simulink model "sampleModel295"  (R2021b)
settings: Solver=VariableStepAuto  StartTime=0.0  StopTime=10.0  RelTol=1e-3
undefined symbols (not defined in the file or in its folder): Newton, Raphson
libraries: simulink x10, slpidlib x2
settings Model: Creator=user  LastModifiedBy=user

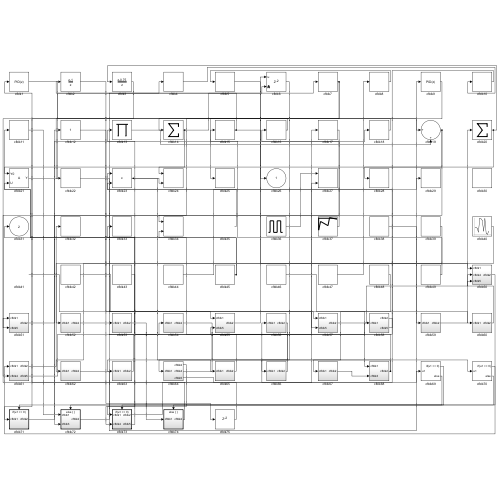
[thumbnail: Simulink's stored preview of the top-level diagram]
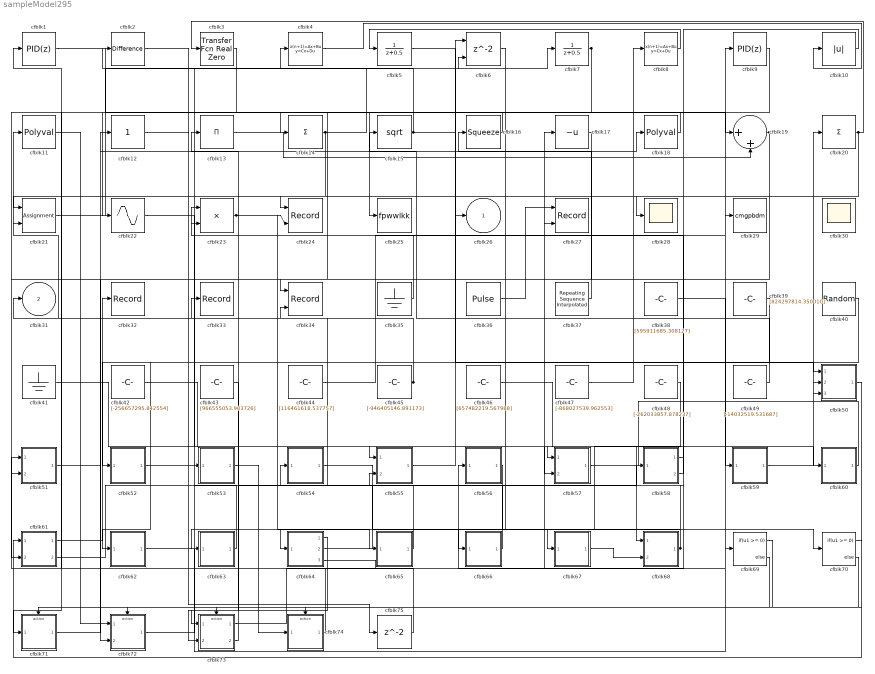
== system sampleModel295 ==
  cfblk1 : slpidlib/PID Controller  Controller=PID  Form=Parallel  TimeDomain=Discrete-time  UseExternalTs=off  SampleTime=1  IntegratorMethod=Forward Euler  FilterMethod=Forward Euler  ControllerParametersSource=internal  P=1  I=1  D=0  UseFilter=on  N=100  TunerSelectOption=Transfer Function Based (PID Tuner App)  InitialConditionSource=internal  InitialConditionForIntegrator=0  InitialConditionForFilter=0  DifferentiatorICPrevScaledInput=0  ExternalReset=none  TrackingMode=off  Kt=1  LimitOutput=off  SatLimitsSource=internal  UpperSaturationLimit=inf  LowerSaturationLimit=-inf  LinearizeAsGain=off  AntiWindupMode=none  Kb=1  POutMin=[]  POutMax=[]  IOutMin=[]  IOutMax=[]  DOutMin=[]  DOutMax=[]  NOutMin=[]  NOutMax=[]  SumOutMin=[]  SumOutMax=[]  SaturationOutMin=[]  SaturationOutMax=[]  PParamMin=[]  PParamMax=[]  IParamMin=[]  IParamMax=[]  DParamMin=[]  DParamMax=[]  NParamMin=[]  NParamMax=[]  KbParamMin=[]  KbParamMax=[]  KtParamMin=[]  KtParamMax=[]  KbOutMin=[]  KbOutMax=[]  KtOutMin=[]  KtOutMax=[]  IntegratorOutMin=[]  IntegratorOutMax=[]  FilterOutMin=[]  FilterOutMax=[]  SumI1OutMin=[]  SumI1OutMax=[]  SumI2OutMin=[]  SumI2OutMax=[]  SumI3OutMin=[]  SumI3OutMax=[]  SumI4OutMin=[]  SumI4OutMax=[]  SumDOutMin=[]  SumDOutMax=[]  DifferentiatorOutMin=[]  DifferentiatorOutMax=[]  FilterDiffOutCoefMin=[]  FilterDiffOutCoefMax=[]  ReciprocalOutMin=[]  ReciprocalOutMax=[]  SumDenOutMin=[]  SumDenOutMax=[]  SumNumOutMin=[]  SumNumOutMax=[]  DivideOutMin=[]  DivideOutMax=[]  UdiffTsProdOutMin=[]  UdiffTsProdOutMax=[]  NTsProdOutMin=[]  NTsProdOutMax=[]  UintegralTsProdOutMin=[]  UintegralTsProdOutMax=[]  UngainTsProdOutMin=[]  UngainTsProdOutMax=[]  IntegratorContinuousStateAttributes=''  IntegratorStateMustResolveToSignalObject=off  IntegratorRTWStateStorageClass=Auto  FilterContinuousStateAttributes=''  FilterStateMustResolveToSignalObject=off  FilterRTWStateStorageClass=Auto  ParallelPVariant=InternalParameters  IdealPVariant=Disabled  IVariant=InternalParameters  DVariant=InternalParameters  IntegratorVariant=Discrete  SatVariant=Disabled  AWVariant=Passthrough  PCopyVariant=Disabled  TRVariant=Disabled  FdbkBlocksVariant=Forward  IdealPFdbkVariant=Disabled  SatFdbkVariant=Disabled  DerivativeFilterVariant=ForwardEulerFilter  NVariant=InternalParameters  NCopyVariant=Disabled  FilterICVariant=InternalICsFilter  IntegratorICVariant=InternalICs  ExternalResetVariant=Disabled  TRSumVariant=Passthrough  SumFdbkVariant=Disabled  SumVariant=Sum_PID  TsampFilterVariant=InternalTs  TsampNgainVariant=Passthrough  TsampIntegralVariant=Passthrough  ExternalSaturationOutDataTypeStr=Inherit: Same as second input
  cfblk10 : Abs
  cfblk11 : Polyval  Coefs=[ +2.081618890e-019, -1.441693666e-014, +4.719686976e-010, -8.536869453e-006, +1.621573104e-001, -8.087801117e+001 ]
  cfblk12 : simulink/Math Operations/Slider Gain  gain=1  low=0  high=2
  cfblk13 : Product  Inputs=*
  cfblk14 : Sum  Inputs=+
  cfblk15 : Sqrt  SaturateOnIntegerOverflow=on
  cfblk16 : Squeeze
  cfblk17 : UnaryMinus
  cfblk18 : Polyval  Coefs=[ +2.081618890e-019, -1.441693666e-014, +4.719686976e-010, -8.536869453e-006, +1.621573104e-001, -8.087801117e+001 ]
  cfblk19 : Sum  Inputs=|++
  cfblk2 : simulink/Discrete/Difference  ICPrevInput=0.0  OutMin=[]  OutMax=[]  OutDataTypeStr=Inherit: Inherit via back propagation  OutDataType=fixdt(1, 16)  OutScaling=2^-10  DoSatur=off
  cfblk20 : Sum  Inputs=+
  cfblk21 : Assignment  DiagnosticForDimensions=Warning  IndexOptions=Index vector (dialog)  Indices=1  OutputSizes=1
  cfblk22 : Sin  TimeSource=Use external signal  SampleTime=0
  cfblk23 : Product  Inputs=**
  cfblk24 : Record  FileSettingsInternal="{\"entries\":[{\"content\":{\"excelSettings\":{\"content\":{},\"type\":\"Streamout.ExcelSettings\"}},\"type\":\"Streamout.FileSettingStorage\",\"uuid\":\"e644294e-47c8-4157-a70f-b86bf0f91ce5\"}],\"packageUris\":[\"http://schema.mathworks.com/mf0/streamout_blocks/R2020a\"],\"version\":\"1.0\"}"  Layout=[1 1]  SignalsInternal="{\"entries\":[{\"content\":{\"signals\":[{\"content\":{\"blockPath\":[\"sampleModel295/cfblk24\"],\"channel\":[],\"dimensions\":[1],\"domain\":\"sampleModel295/cfblk24\",\"lineColor\":\"#a2142f\",\"plots\":[1],\"port\":1,\"sid\":[\"\"],\"signalID\":12729,\"signalName\":\"cfblk14\"},\"type\":\"RecordBlkView.Signal\",\"uuid\":\"f10aec68-513e-477d-a584-377b7a0421ce\"},{\"content\":{\"blockPath\":[\"sampleModel295/cfblk24\"],\"channel\":[],\"dimensions\":[1,1],\"domain\":\"sampleModel295/cfblk24\",\"lineColor\":\"#139fff\",\"plots\":[1],\"port\":2,\"sid\":[\"\"],\"signalID\":12733,\"signalName\":\"cfblk23\"},\"type\":\"RecordBlkView.Signal\",\"uuid\":\"9a725780-6232-41e5-9a59-fff5a766301b\"}]},\"type\":\"RecordBlkView.InputSignals\",\"uuid\":\"3815a519-980c-4b72-ad09-c02e00f9a3ac\"}],\"packageUris\":[\"http://schema.mathworks.com/mf0/streamout_blocks/R2020a\"],\"version\":\"1.0\"}"  VisualizationBindings="{\"xyplotplugin\":{\"info\":[{\"series\":[{\"bindingParametersList\":[{\"parameter\":\"X-Axis\",\"signalID\":12729,\"signalName\":\"cfblk14\"},{\"parameter\":\"Y-Axis\",\"signalID\":12733,\"signalName\":\"cfblk23\"}],\"seriesID\":57202}],\"subplotID\":1}]}}"  CompatibilityTag=XY
  cfblk25 : ToWorkspace  VariableName=fpwwlkk  SaveFormat=Timeseries  SampleTime=-1
  cfblk27 : Record  FileSettingsInternal="{\"entries\":[{\"content\":{\"excelSettings\":{\"content\":{},\"type\":\"Streamout.ExcelSettings\"}},\"type\":\"Streamout.FileSettingStorage\",\"uuid\":\"b7e32862-4def-4129-82f2-dd9595ad73df\"}],\"packageUris\":[\"http://schema.mathworks.com/mf0/streamout_blocks/R2020a\"],\"version\":\"1.0\"}"  Layout=[1 1]  SignalsInternal="{\"entries\":[{\"content\":{\"signals\":[{\"content\":{\"blockPath\":[\"sampleModel295/cfblk27\"],\"channel\":[],\"dimensions\":[1],\"domain\":\"sampleModel295/cfblk27\",\"lineColor\":\"#a2142f\",\"plots\":[1],\"port\":1,\"sid\":[\"\"],\"signalID\":12737,\"signalName\":\"cfblk36\"},\"type\":\"RecordBlkView.Signal\",\"uuid\":\"85d272bf-6785-403c-95ae-8b25dcc783db\"},{\"content\":{\"blockPath\":[\"sampleModel295/cfblk27\"],\"channel\":[],\"dimensions\":[1],\"domain\":\"sampleModel295/cfblk27\",\"lineColor\":\"#139fff\",\"plots\":[1],\"port\":2,\"sid\":[\"\"],\"signalID\":12741,\"signalName\":\"cfblk73:1\"},\"type\":\"RecordBlkView.Signal\",\"uuid\":\"b5cff7ce-ee06-4cac-90c4-86c035636aeb\"}]},\"type\":\"RecordBlkView.InputSignals\",\"uuid\":\"7b9cfb08-aa55-403e-a887-71b5e0abc4a4\"}],\"packageUris\":[\"http://schema.mathworks.com/mf0/streamout_blocks/R2020a\"],\"version\":\"1.0\"}"  VisualizationBindings="{\"xyplotplugin\":{\"info\":[{\"series\":[{\"bindingParametersList\":[{\"parameter\":\"X-Axis\",\"signalID\":12737,\"signalName\":\"cfblk36\"},{\"parameter\":\"Y-Axis\",\"signalID\":12741,\"signalName\":\"cfblk73:1\"}],\"seriesID\":37411}],\"subplotID\":1}]}}"  CompatibilityTag=XY
  cfblk28 : Scope
  cfblk29 : ToWorkspace  VariableName=cmgpbdm  SaveFormat=Timeseries  SampleTime=-1
  cfblk3 : simulink/Discrete/Transfer Fcn Real Zero  ZeroZ=0.75  ICPrevInput=0.0  DoSatur=off
      settings: SourceProductBaseCode=SL
  cfblk30 : Scope
      settings: Floating=on
  cfblk32 : Record  FileSettingsInternal="{\"entries\":[{\"content\":{\"excelSettings\":{\"content\":{},\"type\":\"Streamout.ExcelSettings\"}},\"type\":\"Streamout.FileSettingStorage\",\"uuid\":\"9b634011-b706-471f-8d8c-3277855acf29\"}],\"packageUris\":[\"http://schema.mathworks.com/mf0/streamout_blocks/R2020a\"],\"version\":\"1.0\"}"  SignalsInternal="{\"entries\":[{\"content\":{\"signals\":[{\"content\":{\"blockPath\":[\"sampleModel295/cfblk32\"],\"channel\":[],\"dimensions\":[1],\"domain\":\"sampleModel295/cfblk32\",\"lineColor\":\"#a2142f\",\"plots\":[1],\"port\":1,\"sid\":[\"\"],\"signalID\":12745,\"signalName\":\"cfblk61:1\"},\"type\":\"RecordBlkView.Signal\",\"uuid\":\"713a4e37-51c4-4904-a6cc-f5381fe626eb\"}]},\"type\":\"RecordBlkView.InputSignals\",\"uuid\":\"94e50211-0dd7-4ae3-a9db-9c1dd3a17ac5\"}],\"packageUris\":[\"http://schema.mathworks.com/mf0/streamout_blocks/R2020a\"],\"version\":\"1.0\"}"  VisualizationBindings="{\"sparklinesplugin\":{\"info\":[{\"bindingParametersList\":[],\"subplotID\":1}]}}"
  cfblk33 : Record  FileSettingsInternal="{\"entries\":[{\"content\":{\"excelSettings\":{\"content\":{},\"type\":\"Streamout.ExcelSettings\"}},\"type\":\"Streamout.FileSettingStorage\",\"uuid\":\"9bcf9a1a-6272-4e85-9a14-13b62b86e8eb\"}],\"packageUris\":[\"http://schema.mathworks.com/mf0/streamout_blocks/R2020a\"],\"version\":\"1.0\"}"  SignalsInternal="{\"entries\":[{\"content\":{\"signals\":[{\"content\":{\"blockPath\":[\"sampleModel295/cfblk33\"],\"channel\":[],\"dimensions\":[1,1],\"domain\":\"sampleModel295/cfblk33\",\"lineColor\":\"#139fff\",\"plots\":[1],\"port\":1,\"sid\":[\"\"],\"signalID\":12749,\"signalName\":\"cfblk65\"},\"type\":\"RecordBlkView.Signal\",\"uuid\":\"4cbff2d7-f26b-4c35-8c5f-df1d9d9f7d13\"}]},\"type\":\"RecordBlkView.InputSignals\",\"uuid\":\"b3f169fd-622d-4759-a4e5-6eade6133a40\"}],\"packageUris\":[\"http://schema.mathworks.com/mf0/streamout_blocks/R2020a\"],\"version\":\"1.0\"}"  VisualizationBindings="{\"sparklinesplugin\":{\"info\":[{\"bindingParametersList\":[],\"subplotID\":1}]}}"
  cfblk34 : Record  FileSettingsInternal="{\"entries\":[{\"content\":{\"excelSettings\":{\"content\":{},\"type\":\"Streamout.ExcelSettings\"}},\"type\":\"Streamout.FileSettingStorage\",\"uuid\":\"ad245534-a126-491f-ae91-c836af0e3ad9\"}],\"packageUris\":[\"http://schema.mathworks.com/mf0/streamout_blocks/R2020a\"],\"version\":\"1.0\"}"  Layout=[1 1]  SignalsInternal="{\"entries\":[{\"content\":{\"signals\":[{\"content\":{\"blockPath\":[\"sampleModel295/cfblk34\"],\"channel\":[],\"dimensions\":[1],\"domain\":\"sampleModel295/cfblk34\",\"lineColor\":\"#a2142f\",\"plots\":[1],\"port\":1,\"sid\":[\"\"],\"signalID\":12753,\"signalName\":\"cfblk7\"},\"type\":\"RecordBlkView.Signal\",\"uuid\":\"bce65451-ca10-46cc-b2c4-c9a99149bc20\"},{\"content\":{\"blockPath\":[\"sampleModel295/cfblk34\"],\"channel\":[],\"dimensions\":[1,1],\"domain\":\"sampleModel295/cfblk34\",\"lineColor\":\"#139fff\",\"plots\":[1],\"port\":2,\"sid\":[\"\"],\"signalID\":12757,\"signalName\":\"cfblk68\"},\"type\":\"RecordBlkView.Signal\",\"uuid\":\"bca2518a-e4c1-488f-a659-4f0ad251d5cd\"}]},\"type\":\"RecordBlkView.InputSignals\",\"uuid\":\"252255dc-c8db-4030-b98c-8f428237fd4d\"}],\"packageUris\":[\"http://schema.mathworks.com/mf0/streamout_blocks/R2020a\"],\"version\":\"1.0\"}"  VisualizationBindings="{\"xyplotplugin\":{\"info\":[{\"series\":[{\"bindingParametersList\":[{\"parameter\":\"X-Axis\",\"signalID\":12753,\"signalName\":\"cfblk7\"},{\"parameter\":\"Y-Axis\",\"signalID\":12757,\"signalName\":\"cfblk68\"}],\"seriesID\":47423}],\"subplotID\":1}]}}"  CompatibilityTag=XY
  cfblk35 : Ground
  cfblk36 : DiscretePulseGenerator  PulseType=Time based  Amplitude=[-849674981.811508]  Period=[1552871.382462]  PulseWidth=5  PhaseDelay=[8.000000]
  cfblk37 : simulink/Sources/Repeating Sequence Interpolated  OutValues=[-984002673.050901, -258940035.022713, -628170089.492454, 59276096.145658, -75844292.440838]  TimeValues=[0 0.1 0.5 0.6 1].'  LookUpMeth=Use Input Nearest  tsamp=0.01  OutMin=[]  OutMax=[]  OutDataTypeStr=double  OutputDataTypeScalingMode=double  OutDataType=fixdt(0,8)  OutScaling=2^-10
  cfblk38 : Constant  Value=[595911685.308127]  SampleTime=1
  cfblk39 : Constant  Value=[824297814.350010]  SampleTime=1
  cfblk4 : DiscreteStateSpace
  cfblk40 : RandomNumber  Mean=[37993.970635]  Variance=[6255.361900]  Seed=[560915355.000000]  SampleTime=0.1
  cfblk41 : Ground
  cfblk42 : Constant  Value=[-256657295.842554]  SampleTime=1
  cfblk43 : Constant  Value=[966555053.903726]  SampleTime=1
  cfblk44 : Constant  Value=[116461618.537757]  SampleTime=1
  cfblk45 : Constant  Value=[-946405146.891173]  SampleTime=1
  cfblk46 : Constant  Value=[657482219.567988]  SampleTime=1
  cfblk47 : Constant  Value=[-868027539.962553]  SampleTime=1
  cfblk48 : Constant  Value=[-262033857.878237]  SampleTime=1
  cfblk49 : Constant  Value=[-14032519.531687]  SampleTime=1
  cfblk5 : DiscreteTransferFcn  SampleTime=1
  cfblk50 : Subsystem
  cfblk51 : Subsystem
  cfblk52 : Subsystem
  cfblk53 : Subsystem
  cfblk54 : Subsystem
  cfblk55 : Subsystem
  cfblk56 : Subsystem
  cfblk57 : Subsystem
  cfblk58 : Subsystem
  cfblk59 : Subsystem
  cfblk6 : Delay  ShowEnablePort=on  SampleTime=1
      settings: InputPortMap=u0,e6
  cfblk60 : Subsystem
  cfblk61 : Subsystem
  cfblk62 : Subsystem
  cfblk63 : Subsystem
  cfblk64 : Subsystem
  cfblk65 : Subsystem
  cfblk66 : Subsystem
  cfblk67 : Subsystem
  cfblk68 : Subsystem
  cfblk69 : If  IfExpression=u1 >= 0  SampleTime=1
  cfblk7 : DiscreteTransferFcn  SampleTime=1
  cfblk70 : If  IfExpression=u1 >= 0  SampleTime=1
  cfblk71 : Subsystem  TreatAsAtomicUnit=on
  cfblk72 : Subsystem  TreatAsAtomicUnit=on
  cfblk73 : Subsystem  TreatAsAtomicUnit=on
  cfblk74 : Subsystem  TreatAsAtomicUnit=on
  cfblk75 : Delay  SampleTime=1
  cfblk8 : DiscreteStateSpace
  cfblk9 : slpidlib/PID Controller  Controller=PID  Form=Parallel  TimeDomain=Discrete-time  UseExternalTs=off  SampleTime=1  IntegratorMethod=Forward Euler  FilterMethod=Forward Euler  ControllerParametersSource=internal  P=1  I=1  D=0  UseFilter=on  N=100  TunerSelectOption=Transfer Function Based (PID Tuner App)  InitialConditionSource=internal  InitialConditionForIntegrator=0  InitialConditionForFilter=0  DifferentiatorICPrevScaledInput=0  ExternalReset=none  TrackingMode=off  Kt=1  LimitOutput=off  SatLimitsSource=internal  UpperSaturationLimit=inf  LowerSaturationLimit=-inf  LinearizeAsGain=off  AntiWindupMode=none  Kb=1  POutMin=[]  POutMax=[]  IOutMin=[]  IOutMax=[]  DOutMin=[]  DOutMax=[]  NOutMin=[]  NOutMax=[]  SumOutMin=[]  SumOutMax=[]  SaturationOutMin=[]  SaturationOutMax=[]  PParamMin=[]  PParamMax=[]  IParamMin=[]  IParamMax=[]  DParamMin=[]  DParamMax=[]  NParamMin=[]  NParamMax=[]  KbParamMin=[]  KbParamMax=[]  KtParamMin=[]  KtParamMax=[]  KbOutMin=[]  KbOutMax=[]  KtOutMin=[]  KtOutMax=[]  IntegratorOutMin=[]  IntegratorOutMax=[]  FilterOutMin=[]  FilterOutMax=[]  SumI1OutMin=[]  SumI1OutMax=[]  SumI2OutMin=[]  SumI2OutMax=[]  SumI3OutMin=[]  SumI3OutMax=[]  SumI4OutMin=[]  SumI4OutMax=[]  SumDOutMin=[]  SumDOutMax=[]  DifferentiatorOutMin=[]  DifferentiatorOutMax=[]  FilterDiffOutCoefMin=[]  FilterDiffOutCoefMax=[]  ReciprocalOutMin=[]  ReciprocalOutMax=[]  SumDenOutMin=[]  SumDenOutMax=[]  SumNumOutMin=[]  SumNumOutMax=[]  DivideOutMin=[]  DivideOutMax=[]  UdiffTsProdOutMin=[]  UdiffTsProdOutMax=[]  NTsProdOutMin=[]  NTsProdOutMax=[]  UintegralTsProdOutMin=[]  UintegralTsProdOutMax=[]  UngainTsProdOutMin=[]  UngainTsProdOutMax=[]  IntegratorContinuousStateAttributes=''  IntegratorStateMustResolveToSignalObject=off  IntegratorRTWStateStorageClass=Auto  FilterContinuousStateAttributes=''  FilterStateMustResolveToSignalObject=off  FilterRTWStateStorageClass=Auto  ParallelPVariant=InternalParameters  IdealPVariant=Disabled  IVariant=InternalParameters  DVariant=InternalParameters  IntegratorVariant=Discrete  SatVariant=Disabled  AWVariant=Passthrough  PCopyVariant=Disabled  TRVariant=Disabled  FdbkBlocksVariant=Forward  IdealPFdbkVariant=Disabled  SatFdbkVariant=Disabled  DerivativeFilterVariant=ForwardEulerFilter  NVariant=InternalParameters  NCopyVariant=Disabled  FilterICVariant=InternalICsFilter  IntegratorICVariant=InternalICs  ExternalResetVariant=Disabled  TRSumVariant=Passthrough  SumFdbkVariant=Disabled  SumVariant=Sum_PID  TsampFilterVariant=InternalTs  TsampNgainVariant=Passthrough  TsampIntegralVariant=Passthrough  ExternalSaturationOutDataTypeStr=Inherit: Same as second input
  cfblk26 : Outport
  cfblk31 : Outport  Port=2
  wires:
  cfblk11/1 -> cfblk72/1(cfblk1)
  cfblk36/1 -> cfblk27/1
  cfblk61/1(cfblk2) -> cfblk32/1
  cfblk53/1(cfblk2) -> cfblk74/1(cfblk1)
  cfblk63/1(cfblk2) -> cfblk7/1
  cfblk37/1 -> cfblk16/1
  cfblk22/1 -> cfblk57/1(cfblk1)
  cfblk21/1 -> cfblk4/1
  cfblk62/1(cfblk2) -> cfblk9/1
  cfblk46/1 -> cfblk68/1(cfblk1)
  cfblk61/2(cfblk5) -> cfblk54/1(cfblk1)
  cfblk3/1 -> cfblk22/1
  cfblk10/1 -> cfblk56/1(cfblk1)
  cfblk52/1(cfblk2) -> cfblk53/1(cfblk1)
  cfblk16/1 -> cfblk25/1
  cfblk60/1(cfblk2) -> cfblk20/1
  cfblk8/1 -> cfblk5/1
  cfblk4/1 -> cfblk10/1
  cfblk40/1 -> cfblk52/1(cfblk1)
  cfblk5/1 -> cfblk26/1
  cfblk15/1 -> cfblk50/1(cfblk1), cfblk2/1
  cfblk51/1(cfblk2) -> cfblk12/1
  cfblk67/1(cfblk2) -> cfblk68/2(cfblk3)
  cfblk14/1 -> cfblk24/1, cfblk6/2
  cfblk72/1(cfblk2) -> cfblk17/1
  cfblk66/1(cfblk2) -> cfblk13/1
  cfblk59/1(cfblk2) -> cfblk50/2(cfblk4)
  cfblk71/1(cfblk2) -> cfblk18/1
  cfblk65/1(cfblk2) -> cfblk33/1
  cfblk74/1(cfblk2) -> cfblk1/1
  cfblk41/1 -> cfblk55/1(cfblk1)
  cfblk68/1(cfblk2) -> cfblk64/1(cfblk1), cfblk34/2
  cfblk50/1(cfblk2) -> cfblk61/1(cfblk1)
  cfblk1/1 -> cfblk19/1
  cfblk20/1 -> cfblk3/1, cfblk21/1
  cfblk7/1 -> cfblk71/1(cfblk1), cfblk34/1
  cfblk43/1 -> cfblk73/1(cfblk1)
  cfblk13/1 -> cfblk19/2
  cfblk73/1(cfblk2) -> cfblk27/2
  cfblk57/1(cfblk2) -> cfblk50/3(cfblk5)
  cfblk17/1 -> cfblk51/2(cfblk5)
  cfblk9/1 -> cfblk61/2(cfblk4)
  cfblk6/1 -> cfblk66/1(cfblk1)
  cfblk19/1 -> cfblk72/2(cfblk3), cfblk28/1
  cfblk44/1 -> cfblk29/1
  cfblk47/1 -> cfblk8/1
  cfblk73/2(cfblk5) -> cfblk31/1
  cfblk49/1 -> cfblk15/1
  cfblk18/1 -> cfblk14/1
  cfblk56/1(cfblk2) -> cfblk63/1(cfblk1)
  cfblk55/1(cfblk2) -> cfblk6/1
  cfblk42/1 -> cfblk57/2(cfblk5)
  cfblk35/1 -> cfblk23/1
  cfblk54/1(cfblk2) -> cfblk70/1
  cfblk48/1 -> cfblk67/1(cfblk1)
  cfblk38/1 -> cfblk59/1(cfblk1)
  cfblk2/1 -> cfblk60/1(cfblk1)
  cfblk58/1(cfblk2) -> cfblk55/2(cfblk5)
  cfblk39/1 -> cfblk62/1(cfblk1)
  cfblk45/1 -> cfblk11/1, cfblk21/2
  cfblk23/1 -> cfblk24/2, cfblk65/1(cfblk1)
  cfblk64/1(cfblk2) -> cfblk73/2(cfblk4)
  cfblk64/2(cfblk4) -> cfblk58/1(cfblk1)
  cfblk58/2(cfblk5) -> cfblk23/2
  cfblk64/3(cfblk5) -> cfblk69/1
  cfblk69/1 -> cfblk71/Action
  cfblk69/2 -> cfblk72/Action
  cfblk70/1 -> cfblk73/Action
  cfblk70/2 -> cfblk74/Action
  cfblk12/1 -> cfblk75/1
  cfblk75/1 -> cfblk51/1(cfblk1)

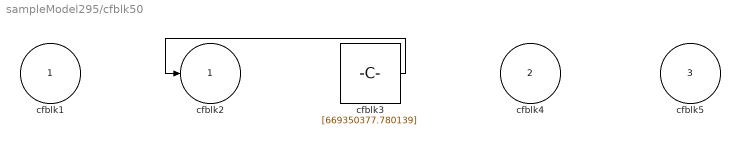
== system sampleModel295/cfblk50 ==
  cfblk1 : Inport
  cfblk4 : Inport  Port=2
  cfblk5 : Inport  Port=3
  cfblk3 : Constant  Value=[669350377.780139]  SampleTime=1
  cfblk2 : Outport
  wires:
  cfblk3/1 -> cfblk2/1

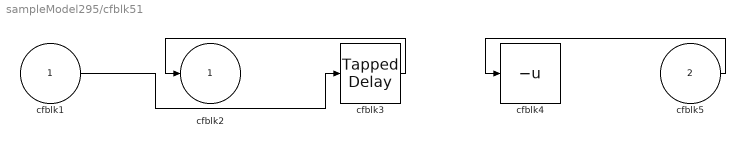
== system sampleModel295/cfblk51 ==
  cfblk1 : Inport
  cfblk5 : Inport  Port=2
  cfblk3 : simulink/Discrete/Tapped Delay  vinit=0.0  samptime=-1  NumDelays=1  DelayOrder=Oldest  includeCurrent=off
  cfblk4 : UnaryMinus
  cfblk2 : Outport
  wires:
  cfblk3/1 -> cfblk2/1
  cfblk1/1 -> cfblk3/1
  cfblk5/1 -> cfblk4/1

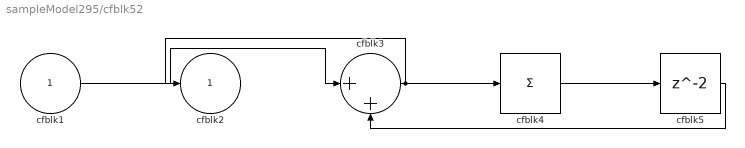
== system sampleModel295/cfblk52 ==
  cfblk1 : Inport
  cfblk3 : Sum  Inputs=|++
  cfblk4 : Sum  Inputs=+
  cfblk5 : Delay  SampleTime=1
  cfblk2 : Outport
  wires:
  cfblk1/1 -> cfblk3/1
  cfblk3/1 -> cfblk2/1, cfblk4/1
  cfblk4/1 -> cfblk5/1
  cfblk5/1 -> cfblk3/2

== system sampleModel295/cfblk53 ==
  cfblk1 : Inport
  cfblk3 : simulink/Discrete/Tapped Delay  vinit=0.0  samptime=-1  NumDelays=1  DelayOrder=Oldest  includeCurrent=off
  cfblk4 : Rounding
  cfblk2 : Outport
  wires:
  cfblk1/1 -> cfblk3/1
  cfblk4/1 -> cfblk2/1
  cfblk3/1 -> cfblk4/1

== system sampleModel295/cfblk54 ==
  cfblk1 : Inport
  cfblk3 : Polyval  Coefs=[ +2.081618890e-019, -1.441693666e-014, +4.719686976e-010, -8.536869453e-006, +1.621573104e-001, -8.087801117e+001 ]
  cfblk2 : Outport
  wires:
  cfblk1/1 -> cfblk2/1, cfblk3/1

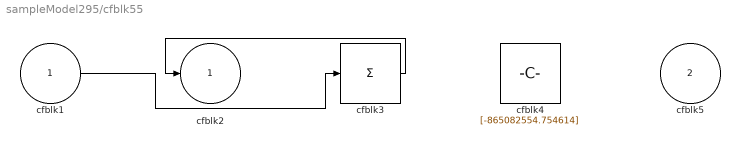
== system sampleModel295/cfblk55 ==
  cfblk1 : Inport
  cfblk5 : Inport  Port=2
  cfblk3 : Sum  Inputs=+
  cfblk4 : Constant  Value=[-865082554.754614]  SampleTime=1
  cfblk2 : Outport
  wires:
  cfblk3/1 -> cfblk2/1
  cfblk1/1 -> cfblk3/1

== system sampleModel295/cfblk56 ==
  cfblk1 : Inport
  cfblk3 : Constant  Value=[253467573.492037]  SampleTime=1
  cfblk2 : Outport
  wires:
  cfblk3/1 -> cfblk2/1

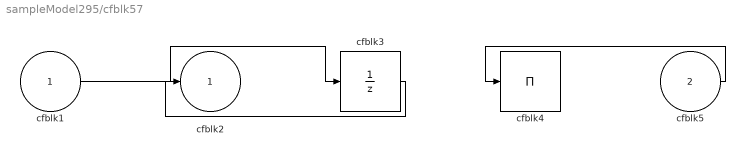
== system sampleModel295/cfblk57 ==
  cfblk1 : Inport
  cfblk5 : Inport  Port=2
  cfblk3 : UnitDelay  HasFrameUpgradeWarning=on
  cfblk4 : Product  Inputs=*
  cfblk2 : Outport
  wires:
  cfblk1/1 -> cfblk3/1
  cfblk3/1 -> cfblk2/1
  cfblk5/1 -> cfblk4/1

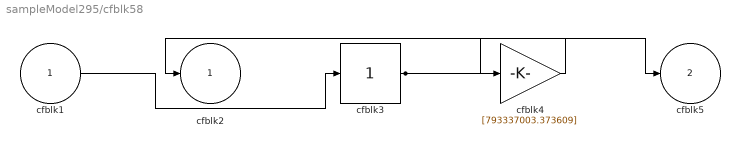
== system sampleModel295/cfblk58 ==
  cfblk1 : Inport
  cfblk3 : simulink/Math Operations/Slider Gain  gain=1  low=0  high=2
  cfblk4 : Gain  Gain=[793337003.373609]
  cfblk2 : Outport
  cfblk5 : Outport  Port=2
  wires:
  cfblk4/1 -> cfblk2/1
  cfblk1/1 -> cfblk3/1
  cfblk3/1 -> cfblk4/1, cfblk5/1

== system sampleModel295/cfblk59 ==
  cfblk1 : Inport
  cfblk3 : ComplexToRealImag
  cfblk4 : Trigonometry
  cfblk2 : Outport
  wires:
  cfblk4/1 -> cfblk2/1
  cfblk1/1 -> cfblk3/1
  cfblk3/1 -> cfblk4/1

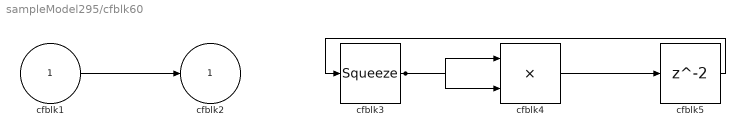
== system sampleModel295/cfblk60 ==
  cfblk1 : Inport
  cfblk3 : Squeeze
  cfblk4 : Product
  cfblk5 : Delay  SampleTime=1
  cfblk2 : Outport
  wires:
  cfblk3/1 -> cfblk4/1, cfblk4/2
  cfblk1/1 -> cfblk2/1
  cfblk4/1 -> cfblk5/1
  cfblk5/1 -> cfblk3/1

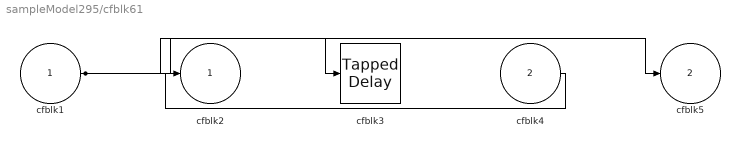
== system sampleModel295/cfblk61 ==
  cfblk1 : Inport
  cfblk4 : Inport  Port=2
  cfblk3 : simulink/Discrete/Tapped Delay  vinit=0.0  samptime=-1  NumDelays=1  DelayOrder=Oldest  includeCurrent=off
  cfblk2 : Outport
  cfblk5 : Outport  Port=2
  wires:
  cfblk1/1 -> cfblk5/1, cfblk3/1
  cfblk4/1 -> cfblk2/1

== system sampleModel295/cfblk62 ==
  cfblk1 : Inport
  cfblk3 : simulink/Math Operations/MinMax Running Resettable  Function=min  vinit=0.0
  cfblk2 : Outport
  wires:
  cfblk3/1 -> cfblk2/1
  cfblk1/1 -> cfblk3/1, cfblk3/2

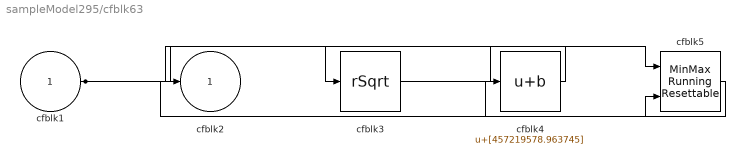
== system sampleModel295/cfblk63 ==
  cfblk1 : Inport
  cfblk3 : Sqrt  Operator=rSqrt  AlgorithmType=Newton-Raphson  SaturateOnIntegerOverflow=on
  cfblk4 : Bias  Bias=[457219578.963745]
  cfblk5 : simulink/Math Operations/MinMax Running Resettable  Function=min  vinit=0.0
  cfblk2 : Outport
  wires:
  cfblk1/1 -> cfblk3/1, cfblk5/2
  cfblk3/1 -> cfblk5/1
  cfblk5/1 -> cfblk4/1
  cfblk4/1 -> cfblk2/1

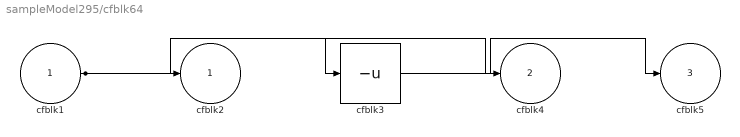
== system sampleModel295/cfblk64 ==
  cfblk1 : Inport
  cfblk3 : UnaryMinus
  cfblk2 : Outport
  cfblk4 : Outport  Port=2
  cfblk5 : Outport  Port=3
  wires:
  cfblk3/1 -> cfblk5/1
  cfblk1/1 -> cfblk4/1, cfblk3/1, cfblk2/1

== system sampleModel295/cfblk65 ==
  cfblk1 : Inport
  cfblk3 : DiscreteStateSpace
  cfblk4 : Rounding
  cfblk5 : Sum  Inputs=+-
  cfblk2 : Outport
  wires:
  cfblk1/1 -> cfblk3/1
  cfblk3/1 -> cfblk5/1, cfblk4/1
  cfblk4/1 -> cfblk5/2
  cfblk5/1 -> cfblk2/1

== system sampleModel295/cfblk66 ==
  cfblk1 : Inport
  cfblk3 : Squeeze
  cfblk2 : Outport
  wires:
  cfblk1/1 -> cfblk3/1
  cfblk3/1 -> cfblk2/1

== system sampleModel295/cfblk67 ==
  cfblk1 : Inport
  cfblk3 : PermuteDimensions
  cfblk2 : Outport
  wires:
  cfblk1/1 -> cfblk3/1
  cfblk3/1 -> cfblk2/1

== system sampleModel295/cfblk68 ==
  cfblk1 : Inport
  cfblk3 : Inport  Port=2
  cfblk2 : Outport
  wires:
  cfblk3/1 -> cfblk2/1

== system sampleModel295/cfblk71 ==
  cfblk1 : Inport
  Action Port : ActionPort  ActionPortLabel=if(u1 >= 0)
  cfblk3 : Delay  ShowEnablePort=on
      settings: InputPortMap=u0,e6
  cfblk2 : Outport
  wires:
  cfblk1/1 -> cfblk3/1, cfblk3/2
  cfblk3/1 -> cfblk2/1

== system sampleModel295/cfblk72 ==
  cfblk1 : Inport
  cfblk3 : Inport  Port=2
  Action Port : ActionPort  ActionPortLabel=else
  cfblk2 : Outport
  wires:
  cfblk1/1 -> cfblk2/1

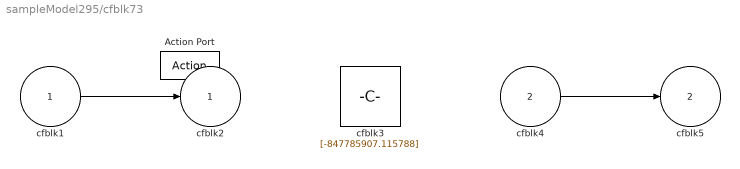
== system sampleModel295/cfblk73 ==
  cfblk1 : Inport
  cfblk4 : Inport  Port=2
  Action Port : ActionPort  ActionPortLabel=if(u1 >= 0)
  cfblk3 : Constant  Value=[-847785907.115788]  SampleTime=1
  cfblk2 : Outport
  cfblk5 : Outport  Port=2
  wires:
  cfblk1/1 -> cfblk2/1
  cfblk4/1 -> cfblk5/1

== system sampleModel295/cfblk74 ==
  cfblk1 : Inport
  Action Port : ActionPort  ActionPortLabel=else
  cfblk3 : Constant  Value=[-704777836.625596]  SampleTime=1
  cfblk2 : Outport
  wires:
  cfblk1/1 -> cfblk2/1
